simulink model "IEEE123bus_v2019b_Discrete_ZIPload"  (R2019b)
settings: Solver=ode4  StartTime=0.0  StopTime=5  FixedStep=Ts  MaxStep=1e-4  RelTol=1e-3
InitFcn:
  | a=1; % Loading Factor
  | Ts=50e-6;
  | % phase to sequence conversion of RXB matrices
  | c=1*exp(sqrt(-1)*(120*pi/180));
  | T=[1 1 1;1 c*c c;1 c c*c];
  | Tinv=1/3*[1 1 1;1 c c*c;1 c*c c];
  | 
  | % Simulation data for the IEEE 123 Node Test Feeder model
  | mi2km = 1.60934;%  miles to km conversion
  | ft2km = 0.0003048; % feet to km conversion
  | ms2F = 1*1e-6/(2*pi*60);% microsiemens to Farads conversion
  | 
  | %% Configuration 1
  | % Series Resitance and Reactance - ohm/mile
  | R_1 = [0.4576 0.1560 0.1535;0.1560 0.4666 0.1580;0.1535 0.1580 0.4615];
  | X_1 = [1.0780 0.5017 0.3849;0.5017 1.0482 0.4236;0.3849 0.4236 1.0651];
  | % charging susceptance - microsiemens/mile
  | B_1 = [5.6765 -1.8319 -0.6982;-1.8319 5.9809 -1.1645;-0.6982 -1.1645 5.3971];
  | 
  | R_1 = R_1/mi2km;
  | Rseq=Tinv*R_1*T;
  | R1_1=Rseq(2,2);R0_1=Rseq(1,1);
  | 
  | L_1 = (X_1/(2*pi*60))/mi2km;
  | Lseq=Tinv*L_1*T;
  | L1_1=Lseq(2,2);L0_1=Lseq(1,1);
  | 
  | C_1 =(B_1*ms2F)/mi2km;
  | Cseq=Tinv*C_1*T;
  | C1_1=Cseq(2,2);C0_1=Cseq(1,1);
  | %% Configuration 2 - series reactance - ohm/mile
  | R_2 = [0.4666 0.1580 0.1560;0.1580 0.4615 0.1535;0.1560 0.1535 0.4576];
  | X_2 = [1.0482 0.4236 0.5017;0.4236 1.0651 0.3849;0.5017 0.3849 1.0780];
  | % charging susceptance - microsiemens/mile
  | B_2 = [5.9809 -1.1645 -1.8319;-1.1645 5.3971 -0.6982;-1.8319 -0.6982 5.6765];
  | 
  | R_2 = R_2/mi2km;
  | Rseq=Tinv*R_2*T;
  | R1_2=Rseq(2,2);R0_2=Rseq(1,1);
  | 
  | L_2 = (X_2/(2*pi*60))/mi2km;
  | Lseq=Tinv*L_2*T;
  | L1_2=Lseq(2,2);L0_2=Lseq(1,1);
  | 
  | C_2 =(B_2*ms2F)/mi2km;
  | Cseq=Tinv*C_2*T;
  | C1_2=Cseq(2,2);C0_2=Cseq(1,1);
  | %% Configuration 3 - series reactance - ohm/mile
  | R_3 = [0.4615 0.1535 0.1580;0.1535 0.4576 0.1560;0.1580 0.1560 0.4666];
  | X_3 = [1.0651 0.3849 0.4236;0.3849 1.0780 0.5017;0.4236 0.5017 1.0482];
  | % charging susceptance - microsiemens/mile
  | B_3 = [5.3971 -0.6982 -1.1645;-0.6982 5.6765 -1.8319; -1.1645 -1.8319 5.9809];
  | 
  | R_3 = R_3/mi2km;
  | Rseq=Tinv*R_3*T;
  | R1_3=Rseq(2,2);R0_3=Rseq(1,1);
  | 
  | L_3 = (X_3/(2*pi*60))/mi2km;
  | Lseq=Tinv*L_3*T;
  | L1_3=Lseq(2,2);L0_3=Lseq(1,1);
  | ... (+157 lines)
undefined symbols (not defined in the file): D1, Delta, find_system
libraries: powerlib x971, powerlib_meascontrol x294
(part 14 of 14)

== matlab function IEEE123bus_v2019b_Discrete_ZIPload/55 Y Z/Embedded MATLAB Function ==
  data: Iinjinst output; Vmeas input; LoadType parameter; Vnom parameter; Pnom parameter; Qnom parameter; Vlim parameter; fnom parameter; clock input; Ddel input
%Single Phase ZIP Load
%Author: Arun Suresh, University of North Carolina, Charlotte
%Iinj=((Pnom+jQnom)/Vmeas)'
function Iinjinst = InjectedCurrent(Vmeas,LoadType,Vnom,Pnom,Qnom,Vlim,fnom,clock,Ddel)
% Calculate Pl and Ql.
%  Vmeas=1.2303e+03 + 1.9328e+03i;
Kz=0;Ki=0;Kp=0;
Vk=(abs(Vmeas)/Vnom);%(Vmeas/Vnom)
switch LoadType  % 1 for Constant Z, 2 for Constant I and 3 for Constant P, 
    case 1
        Kz=1;
    case 2
        if Vk >= Vlim % convert to Constant Z load due to voltage violation
            Ki=1;
        else
            Kz=1;
        end
    case 3
        if Vk >= Vlim % convert to Constant Z load due to voltage violation
           Kp=1;
        else
            Kz=1;
        end          
 
end
Pl=Pnom *((Kz*Vk*Vk)+(Ki*Vk)+(Kp));
Ql=Qnom *((Kz*Vk*Vk)+(Ki*Vk)+(Kp));
% Net Injected Curent.
% j=sqrt(-1);
Iinj = conj((Pl+j*Ql)/Vmeas);
Iinjinst =abs(Iinj)*sqrt(2)*sin(2*fnom*pi*clock + angle(Iinj)+Ddel);
yt=Iinj;

== matlab function IEEE123bus_v2019b_Discrete_ZIPload/64 Y I/Embedded MATLAB Function ==
  data: Iinjinst output; Vmeas input; LoadType parameter; Vnom parameter; Pnom parameter; Qnom parameter; Vlim parameter; fnom parameter; clock input; Ddel input
%Single Phase ZIP Load
%Author: Arun Suresh, University of North Carolina, Charlotte
%Iinj=((Pnom+jQnom)/Vmeas)'
function Iinjinst = InjectedCurrent(Vmeas,LoadType,Vnom,Pnom,Qnom,Vlim,fnom,clock,Ddel)
% Calculate Pl and Ql.
%  Vmeas=1.2303e+03 + 1.9328e+03i;
Kz=0;Ki=0;Kp=0;
Vk=(abs(Vmeas)/Vnom);%(Vmeas/Vnom)
switch LoadType  % 1 for Constant Z, 2 for Constant I and 3 for Constant P, 
    case 1
        Kz=1;
    case 2
        if Vk >= Vlim % convert to Constant Z load due to voltage violation
            Ki=1;
        else
            Kz=1;
        end
    case 3
        if Vk >= Vlim % convert to Constant Z load due to voltage violation
           Kp=1;
        else
            Kz=1;
        end          
 
end
Pl=Pnom *((Kz*Vk*Vk)+(Ki*Vk)+(Kp));
Ql=Qnom *((Kz*Vk*Vk)+(Ki*Vk)+(Kp));
% Net Injected Curent.
% j=sqrt(-1);
Iinj = conj((Pl+j*Ql)/Vmeas);
Iinjinst =abs(Iinj)*sqrt(2)*sin(2*fnom*pi*clock + angle(Iinj)+Ddel);
yt=Iinj;

== matlab function IEEE123bus_v2019b_Discrete_ZIPload/66 Y PQ/Embedded MATLAB Function ==
  data: Iinjinst output; Vmeas input; LoadType parameter; Vnom parameter; Pnom parameter; Qnom parameter; Vlim parameter; fnom parameter; clock input; Ddel input
%Single Phase ZIP Load
%Author: Arun Suresh, University of North Carolina, Charlotte
%Iinj=((Pnom+jQnom)/Vmeas)'
function Iinjinst = InjectedCurrent(Vmeas,LoadType,Vnom,Pnom,Qnom,Vlim,fnom,clock,Ddel)
% Calculate Pl and Ql.
%  Vmeas=1.2303e+03 + 1.9328e+03i;
Kz=0;Ki=0;Kp=0;
Vk=(abs(Vmeas)/Vnom);%(Vmeas/Vnom)
switch LoadType  % 1 for Constant Z, 2 for Constant I and 3 for Constant P, 
    case 1
        Kz=1;
    case 2
        if Vk >= Vlim % convert to Constant Z load due to voltage violation
            Ki=1;
        else
            Kz=1;
        end
    case 3
        if Vk >= Vlim % convert to Constant Z load due to voltage violation
           Kp=1;
        else
            Kz=1;
        end          
 
end
Pl=Pnom *((Kz*Vk*Vk)+(Ki*Vk)+(Kp));
Ql=Qnom *((Kz*Vk*Vk)+(Ki*Vk)+(Kp));
% Net Injected Curent.
% j=sqrt(-1);
Iinj = conj((Pl+j*Ql)/Vmeas);
Iinjinst =abs(Iinj)*sqrt(2)*sin(2*fnom*pi*clock + angle(Iinj)+Ddel);
yt=Iinj;

== matlab function IEEE123bus_v2019b_Discrete_ZIPload/96 Y PQ/Embedded MATLAB Function ==
  data: Iinjinst output; Vmeas input; LoadType parameter; Vnom parameter; Pnom parameter; Qnom parameter; Vlim parameter; fnom parameter; clock input; Ddel input
%Single Phase ZIP Load
%Author: Arun Suresh, University of North Carolina, Charlotte
%Iinj=((Pnom+jQnom)/Vmeas)'
function Iinjinst = InjectedCurrent(Vmeas,LoadType,Vnom,Pnom,Qnom,Vlim,fnom,clock,Ddel)
% Calculate Pl and Ql.
%  Vmeas=1.2303e+03 + 1.9328e+03i;
Kz=0;Ki=0;Kp=0;
Vk=(abs(Vmeas)/Vnom);%(Vmeas/Vnom)
switch LoadType  % 1 for Constant Z, 2 for Constant I and 3 for Constant P, 
    case 1
        Kz=1;
    case 2
        if Vk >= Vlim % convert to Constant Z load due to voltage violation
            Ki=1;
        else
            Kz=1;
        end
    case 3
        if Vk >= Vlim % convert to Constant Z load due to voltage violation
           Kp=1;
        else
            Kz=1;
        end          
 
end
Pl=Pnom *((Kz*Vk*Vk)+(Ki*Vk)+(Kp));
Ql=Qnom *((Kz*Vk*Vk)+(Ki*Vk)+(Kp));
% Net Injected Curent.
% j=sqrt(-1);
Iinj = conj((Pl+j*Ql)/Vmeas);
Iinjinst =abs(Iinj)*sqrt(2)*sin(2*fnom*pi*clock + angle(Iinj)+Ddel);
yt=Iinj;

== matlab function IEEE123bus_v2019b_Discrete_ZIPload/95 Y PQ/Embedded MATLAB Function ==
  data: Iinjinst output; Vmeas input; LoadType parameter; Vnom parameter; Pnom parameter; Qnom parameter; Vlim parameter; fnom parameter; clock input; Ddel input
%Single Phase ZIP Load
%Author: Arun Suresh, University of North Carolina, Charlotte
%Iinj=((Pnom+jQnom)/Vmeas)'
function Iinjinst = InjectedCurrent(Vmeas,LoadType,Vnom,Pnom,Qnom,Vlim,fnom,clock,Ddel)
% Calculate Pl and Ql.
%  Vmeas=1.2303e+03 + 1.9328e+03i;
Kz=0;Ki=0;Kp=0;
Vk=(abs(Vmeas)/Vnom);%(Vmeas/Vnom)
switch LoadType  % 1 for Constant Z, 2 for Constant I and 3 for Constant P, 
    case 1
        Kz=1;
    case 2
        if Vk >= Vlim % convert to Constant Z load due to voltage violation
            Ki=1;
        else
            Kz=1;
        end
    case 3
        if Vk >= Vlim % convert to Constant Z load due to voltage violation
           Kp=1;
        else
            Kz=1;
        end          
 
end
Pl=Pnom *((Kz*Vk*Vk)+(Ki*Vk)+(Kp));
Ql=Qnom *((Kz*Vk*Vk)+(Ki*Vk)+(Kp));
% Net Injected Curent.
% j=sqrt(-1);
Iinj = conj((Pl+j*Ql)/Vmeas);
Iinjinst =abs(Iinj)*sqrt(2)*sin(2*fnom*pi*clock + angle(Iinj)+Ddel);
yt=Iinj;

== matlab function IEEE123bus_v2019b_Discrete_ZIPload/111 Y PQ/Embedded MATLAB Function ==
  data: Iinjinst output; Vmeas input; LoadType parameter; Vnom parameter; Pnom parameter; Qnom parameter; Vlim parameter; fnom parameter; clock input; Ddel input
%Single Phase ZIP Load
%Author: Arun Suresh, University of North Carolina, Charlotte
%Iinj=((Pnom+jQnom)/Vmeas)'
function Iinjinst = InjectedCurrent(Vmeas,LoadType,Vnom,Pnom,Qnom,Vlim,fnom,clock,Ddel)
% Calculate Pl and Ql.
%  Vmeas=1.2303e+03 + 1.9328e+03i;
Kz=0;Ki=0;Kp=0;
Vk=(abs(Vmeas)/Vnom);%(Vmeas/Vnom)
switch LoadType  % 1 for Constant Z, 2 for Constant I and 3 for Constant P, 
    case 1
        Kz=1;
    case 2
        if Vk >= Vlim % convert to Constant Z load due to voltage violation
            Ki=1;
        else
            Kz=1;
        end
    case 3
        if Vk >= Vlim % convert to Constant Z load due to voltage violation
           Kp=1;
        else
            Kz=1;
        end          
 
end
Pl=Pnom *((Kz*Vk*Vk)+(Ki*Vk)+(Kp));
Ql=Qnom *((Kz*Vk*Vk)+(Ki*Vk)+(Kp));
% Net Injected Curent.
% j=sqrt(-1);
Iinj = conj((Pl+j*Ql)/Vmeas);
Iinjinst =abs(Iinj)*sqrt(2)*sin(2*fnom*pi*clock + angle(Iinj)+Ddel);
yt=Iinj;

== matlab function IEEE123bus_v2019b_Discrete_ZIPload/109 Y PQ/Embedded MATLAB Function ==
  data: Iinjinst output; Vmeas input; LoadType parameter; Vnom parameter; Pnom parameter; Qnom parameter; Vlim parameter; fnom parameter; clock input; Ddel input
%Single Phase ZIP Load
%Author: Arun Suresh, University of North Carolina, Charlotte
%Iinj=((Pnom+jQnom)/Vmeas)'
function Iinjinst = InjectedCurrent(Vmeas,LoadType,Vnom,Pnom,Qnom,Vlim,fnom,clock,Ddel)
% Calculate Pl and Ql.
%  Vmeas=1.2303e+03 + 1.9328e+03i;
Kz=0;Ki=0;Kp=0;
Vk=(abs(Vmeas)/Vnom);%(Vmeas/Vnom)
switch LoadType  % 1 for Constant Z, 2 for Constant I and 3 for Constant P, 
    case 1
        Kz=1;
    case 2
        if Vk >= Vlim % convert to Constant Z load due to voltage violation
            Ki=1;
        else
            Kz=1;
        end
    case 3
        if Vk >= Vlim % convert to Constant Z load due to voltage violation
           Kp=1;
        else
            Kz=1;
        end          
 
end
Pl=Pnom *((Kz*Vk*Vk)+(Ki*Vk)+(Kp));
Ql=Qnom *((Kz*Vk*Vk)+(Ki*Vk)+(Kp));
% Net Injected Curent.
% j=sqrt(-1);
Iinj = conj((Pl+j*Ql)/Vmeas);
Iinjinst =abs(Iinj)*sqrt(2)*sin(2*fnom*pi*clock + angle(Iinj)+Ddel);
yt=Iinj;

== matlab function IEEE123bus_v2019b_Discrete_ZIPload/114 Y PQ/Embedded MATLAB Function ==
  data: Iinjinst output; Vmeas input; LoadType parameter; Vnom parameter; Pnom parameter; Qnom parameter; Vlim parameter; fnom parameter; clock input; Ddel input
%Single Phase ZIP Load
%Author: Arun Suresh, University of North Carolina, Charlotte
%Iinj=((Pnom+jQnom)/Vmeas)'
function Iinjinst = InjectedCurrent(Vmeas,LoadType,Vnom,Pnom,Qnom,Vlim,fnom,clock,Ddel)
% Calculate Pl and Ql.
%  Vmeas=1.2303e+03 + 1.9328e+03i;
Kz=0;Ki=0;Kp=0;
Vk=(abs(Vmeas)/Vnom);%(Vmeas/Vnom)
switch LoadType  % 1 for Constant Z, 2 for Constant I and 3 for Constant P, 
    case 1
        Kz=1;
    case 2
        if Vk >= Vlim % convert to Constant Z load due to voltage violation
            Ki=1;
        else
            Kz=1;
        end
    case 3
        if Vk >= Vlim % convert to Constant Z load due to voltage violation
           Kp=1;
        else
            Kz=1;
        end          
 
end
Pl=Pnom *((Kz*Vk*Vk)+(Ki*Vk)+(Kp));
Ql=Qnom *((Kz*Vk*Vk)+(Ki*Vk)+(Kp));
% Net Injected Curent.
% j=sqrt(-1);
Iinj = conj((Pl+j*Ql)/Vmeas);
Iinjinst =abs(Iinj)*sqrt(2)*sin(2*fnom*pi*clock + angle(Iinj)+Ddel);
yt=Iinj;

== matlab function IEEE123bus_v2019b_Discrete_ZIPload/113 Y Z/Embedded MATLAB Function ==
  data: Iinjinst output; Vmeas input; LoadType parameter; Vnom parameter; Pnom parameter; Qnom parameter; Vlim parameter; fnom parameter; clock input; Ddel input
%Single Phase ZIP Load
%Author: Arun Suresh, University of North Carolina, Charlotte
%Iinj=((Pnom+jQnom)/Vmeas)'
function Iinjinst = InjectedCurrent(Vmeas,LoadType,Vnom,Pnom,Qnom,Vlim,fnom,clock,Ddel)
% Calculate Pl and Ql.
%  Vmeas=1.2303e+03 + 1.9328e+03i;
Kz=0;Ki=0;Kp=0;
Vk=(abs(Vmeas)/Vnom);%(Vmeas/Vnom)
switch LoadType  % 1 for Constant Z, 2 for Constant I and 3 for Constant P, 
    case 1
        Kz=1;
    case 2
        if Vk >= Vlim % convert to Constant Z load due to voltage violation
            Ki=1;
        else
            Kz=1;
        end
    case 3
        if Vk >= Vlim % convert to Constant Z load due to voltage violation
           Kp=1;
        else
            Kz=1;
        end          
 
end
Pl=Pnom *((Kz*Vk*Vk)+(Ki*Vk)+(Kp));
Ql=Qnom *((Kz*Vk*Vk)+(Ki*Vk)+(Kp));
% Net Injected Curent.
% j=sqrt(-1);
Iinj = conj((Pl+j*Ql)/Vmeas);
Iinjinst =abs(Iinj)*sqrt(2)*sin(2*fnom*pi*clock + angle(Iinj)+Ddel);
yt=Iinj;

== matlab function IEEE123bus_v2019b_Discrete_ZIPload/112 Y I/Embedded MATLAB Function ==
  data: Iinjinst output; Vmeas input; LoadType parameter; Vnom parameter; Pnom parameter; Qnom parameter; Vlim parameter; fnom parameter; clock input; Ddel input
%Single Phase ZIP Load
%Author: Arun Suresh, University of North Carolina, Charlotte
%Iinj=((Pnom+jQnom)/Vmeas)'
function Iinjinst = InjectedCurrent(Vmeas,LoadType,Vnom,Pnom,Qnom,Vlim,fnom,clock,Ddel)
% Calculate Pl and Ql.
%  Vmeas=1.2303e+03 + 1.9328e+03i;
Kz=0;Ki=0;Kp=0;
Vk=(abs(Vmeas)/Vnom);%(Vmeas/Vnom)
switch LoadType  % 1 for Constant Z, 2 for Constant I and 3 for Constant P, 
    case 1
        Kz=1;
    case 2
        if Vk >= Vlim % convert to Constant Z load due to voltage violation
            Ki=1;
        else
            Kz=1;
        end
    case 3
        if Vk >= Vlim % convert to Constant Z load due to voltage violation
           Kp=1;
        else
            Kz=1;
        end          
 
end
Pl=Pnom *((Kz*Vk*Vk)+(Ki*Vk)+(Kp));
Ql=Qnom *((Kz*Vk*Vk)+(Ki*Vk)+(Kp));
% Net Injected Curent.
% j=sqrt(-1);
Iinj = conj((Pl+j*Ql)/Vmeas);
Iinjinst =abs(Iinj)*sqrt(2)*sin(2*fnom*pi*clock + angle(Iinj)+Ddel);
yt=Iinj;

== matlab function IEEE123bus_v2019b_Discrete_ZIPload/106 Y PQ/Embedded MATLAB Function ==
  data: Iinjinst output; Vmeas input; LoadType parameter; Vnom parameter; Pnom parameter; Qnom parameter; Vlim parameter; fnom parameter; clock input; Ddel input
%Single Phase ZIP Load
%Author: Arun Suresh, University of North Carolina, Charlotte
%Iinj=((Pnom+jQnom)/Vmeas)'
function Iinjinst = InjectedCurrent(Vmeas,LoadType,Vnom,Pnom,Qnom,Vlim,fnom,clock,Ddel)
% Calculate Pl and Ql.
%  Vmeas=1.2303e+03 + 1.9328e+03i;
Kz=0;Ki=0;Kp=0;
Vk=(abs(Vmeas)/Vnom);%(Vmeas/Vnom)
switch LoadType  % 1 for Constant Z, 2 for Constant I and 3 for Constant P, 
    case 1
        Kz=1;
    case 2
        if Vk >= Vlim % convert to Constant Z load due to voltage violation
            Ki=1;
        else
            Kz=1;
        end
    case 3
        if Vk >= Vlim % convert to Constant Z load due to voltage violation
           Kp=1;
        else
            Kz=1;
        end          
 
end
Pl=Pnom *((Kz*Vk*Vk)+(Ki*Vk)+(Kp));
Ql=Qnom *((Kz*Vk*Vk)+(Ki*Vk)+(Kp));
% Net Injected Curent.
% j=sqrt(-1);
Iinj = conj((Pl+j*Ql)/Vmeas);
Iinjinst =abs(Iinj)*sqrt(2)*sin(2*fnom*pi*clock + angle(Iinj)+Ddel);
yt=Iinj;

== matlab function IEEE123bus_v2019b_Discrete_ZIPload/107 Y PQ/Embedded MATLAB Function ==
  data: Iinjinst output; Vmeas input; LoadType parameter; Vnom parameter; Pnom parameter; Qnom parameter; Vlim parameter; fnom parameter; clock input; Ddel input
%Single Phase ZIP Load
%Author: Arun Suresh, University of North Carolina, Charlotte
%Iinj=((Pnom+jQnom)/Vmeas)'
function Iinjinst = InjectedCurrent(Vmeas,LoadType,Vnom,Pnom,Qnom,Vlim,fnom,clock,Ddel)
% Calculate Pl and Ql.
%  Vmeas=1.2303e+03 + 1.9328e+03i;
Kz=0;Ki=0;Kp=0;
Vk=(abs(Vmeas)/Vnom);%(Vmeas/Vnom)
switch LoadType  % 1 for Constant Z, 2 for Constant I and 3 for Constant P, 
    case 1
        Kz=1;
    case 2
        if Vk >= Vlim % convert to Constant Z load due to voltage violation
            Ki=1;
        else
            Kz=1;
        end
    case 3
        if Vk >= Vlim % convert to Constant Z load due to voltage violation
           Kp=1;
        else
            Kz=1;
        end          
 
end
Pl=Pnom *((Kz*Vk*Vk)+(Ki*Vk)+(Kp));
Ql=Qnom *((Kz*Vk*Vk)+(Ki*Vk)+(Kp));
% Net Injected Curent.
% j=sqrt(-1);
Iinj = conj((Pl+j*Ql)/Vmeas);
Iinjinst =abs(Iinj)*sqrt(2)*sin(2*fnom*pi*clock + angle(Iinj)+Ddel);
yt=Iinj;

== matlab function IEEE123bus_v2019b_Discrete_ZIPload/103 Y PQ/Embedded MATLAB Function ==
  data: Iinjinst output; Vmeas input; LoadType parameter; Vnom parameter; Pnom parameter; Qnom parameter; Vlim parameter; fnom parameter; clock input; Ddel input
%Single Phase ZIP Load
%Author: Arun Suresh, University of North Carolina, Charlotte
%Iinj=((Pnom+jQnom)/Vmeas)'
function Iinjinst = InjectedCurrent(Vmeas,LoadType,Vnom,Pnom,Qnom,Vlim,fnom,clock,Ddel)
% Calculate Pl and Ql.
%  Vmeas=1.2303e+03 + 1.9328e+03i;
Kz=0;Ki=0;Kp=0;
Vk=(abs(Vmeas)/Vnom);%(Vmeas/Vnom)
switch LoadType  % 1 for Constant Z, 2 for Constant I and 3 for Constant P, 
    case 1
        Kz=1;
    case 2
        if Vk >= Vlim % convert to Constant Z load due to voltage violation
            Ki=1;
        else
            Kz=1;
        end
    case 3
        if Vk >= Vlim % convert to Constant Z load due to voltage violation
           Kp=1;
        else
            Kz=1;
        end          
 
end
Pl=Pnom *((Kz*Vk*Vk)+(Ki*Vk)+(Kp));
Ql=Qnom *((Kz*Vk*Vk)+(Ki*Vk)+(Kp));
% Net Injected Curent.
% j=sqrt(-1);
Iinj = conj((Pl+j*Ql)/Vmeas);
Iinjinst =abs(Iinj)*sqrt(2)*sin(2*fnom*pi*clock + angle(Iinj)+Ddel);
yt=Iinj;

== matlab function IEEE123bus_v2019b_Discrete_ZIPload/104 Y PQ/Embedded MATLAB Function ==
  data: Iinjinst output; Vmeas input; LoadType parameter; Vnom parameter; Pnom parameter; Qnom parameter; Vlim parameter; fnom parameter; clock input; Ddel input
%Single Phase ZIP Load
%Author: Arun Suresh, University of North Carolina, Charlotte
%Iinj=((Pnom+jQnom)/Vmeas)'
function Iinjinst = InjectedCurrent(Vmeas,LoadType,Vnom,Pnom,Qnom,Vlim,fnom,clock,Ddel)
% Calculate Pl and Ql.
%  Vmeas=1.2303e+03 + 1.9328e+03i;
Kz=0;Ki=0;Kp=0;
Vk=(abs(Vmeas)/Vnom);%(Vmeas/Vnom)
switch LoadType  % 1 for Constant Z, 2 for Constant I and 3 for Constant P, 
    case 1
        Kz=1;
    case 2
        if Vk >= Vlim % convert to Constant Z load due to voltage violation
            Ki=1;
        else
            Kz=1;
        end
    case 3
        if Vk >= Vlim % convert to Constant Z load due to voltage violation
           Kp=1;
        else
            Kz=1;
        end          
 
end
Pl=Pnom *((Kz*Vk*Vk)+(Ki*Vk)+(Kp));
Ql=Qnom *((Kz*Vk*Vk)+(Ki*Vk)+(Kp));
% Net Injected Curent.
% j=sqrt(-1);
Iinj = conj((Pl+j*Ql)/Vmeas);
Iinjinst =abs(Iinj)*sqrt(2)*sin(2*fnom*pi*clock + angle(Iinj)+Ddel);
yt=Iinj;

== matlab function IEEE123bus_v2019b_Discrete_ZIPload/102 Y PQ/Embedded MATLAB Function ==
  data: Iinjinst output; Vmeas input; LoadType parameter; Vnom parameter; Pnom parameter; Qnom parameter; Vlim parameter; fnom parameter; clock input; Ddel input
%Single Phase ZIP Load
%Author: Arun Suresh, University of North Carolina, Charlotte
%Iinj=((Pnom+jQnom)/Vmeas)'
function Iinjinst = InjectedCurrent(Vmeas,LoadType,Vnom,Pnom,Qnom,Vlim,fnom,clock,Ddel)
% Calculate Pl and Ql.
%  Vmeas=1.2303e+03 + 1.9328e+03i;
Kz=0;Ki=0;Kp=0;
Vk=(abs(Vmeas)/Vnom);%(Vmeas/Vnom)
switch LoadType  % 1 for Constant Z, 2 for Constant I and 3 for Constant P, 
    case 1
        Kz=1;
    case 2
        if Vk >= Vlim % convert to Constant Z load due to voltage violation
            Ki=1;
        else
            Kz=1;
        end
    case 3
        if Vk >= Vlim % convert to Constant Z load due to voltage violation
           Kp=1;
        else
            Kz=1;
        end          
 
end
Pl=Pnom *((Kz*Vk*Vk)+(Ki*Vk)+(Kp));
Ql=Qnom *((Kz*Vk*Vk)+(Ki*Vk)+(Kp));
% Net Injected Curent.
% j=sqrt(-1);
Iinj = conj((Pl+j*Ql)/Vmeas);
Iinjinst =abs(Iinj)*sqrt(2)*sin(2*fnom*pi*clock + angle(Iinj)+Ddel);
yt=Iinj;

== matlab function IEEE123bus_v2019b_Discrete_ZIPload/98 Y PQ/Embedded MATLAB Function ==
  data: Iinjinst output; Vmeas input; LoadType parameter; Vnom parameter; Pnom parameter; Qnom parameter; Vlim parameter; fnom parameter; clock input; Ddel input
%Single Phase ZIP Load
%Author: Arun Suresh, University of North Carolina, Charlotte
%Iinj=((Pnom+jQnom)/Vmeas)'
function Iinjinst = InjectedCurrent(Vmeas,LoadType,Vnom,Pnom,Qnom,Vlim,fnom,clock,Ddel)
% Calculate Pl and Ql.
%  Vmeas=1.2303e+03 + 1.9328e+03i;
Kz=0;Ki=0;Kp=0;
Vk=(abs(Vmeas)/Vnom);%(Vmeas/Vnom)
switch LoadType  % 1 for Constant Z, 2 for Constant I and 3 for Constant P, 
    case 1
        Kz=1;
    case 2
        if Vk >= Vlim % convert to Constant Z load due to voltage violation
            Ki=1;
        else
            Kz=1;
        end
    case 3
        if Vk >= Vlim % convert to Constant Z load due to voltage violation
           Kp=1;
        else
            Kz=1;
        end          
 
end
Pl=Pnom *((Kz*Vk*Vk)+(Ki*Vk)+(Kp));
Ql=Qnom *((Kz*Vk*Vk)+(Ki*Vk)+(Kp));
% Net Injected Curent.
% j=sqrt(-1);
Iinj = conj((Pl+j*Ql)/Vmeas);
Iinjinst =abs(Iinj)*sqrt(2)*sin(2*fnom*pi*clock + angle(Iinj)+Ddel);
yt=Iinj;

== matlab function IEEE123bus_v2019b_Discrete_ZIPload/99 Y PQ/Embedded MATLAB Function ==
  data: Iinjinst output; Vmeas input; LoadType parameter; Vnom parameter; Pnom parameter; Qnom parameter; Vlim parameter; fnom parameter; clock input; Ddel input
%Single Phase ZIP Load
%Author: Arun Suresh, University of North Carolina, Charlotte
%Iinj=((Pnom+jQnom)/Vmeas)'
function Iinjinst = InjectedCurrent(Vmeas,LoadType,Vnom,Pnom,Qnom,Vlim,fnom,clock,Ddel)
% Calculate Pl and Ql.
%  Vmeas=1.2303e+03 + 1.9328e+03i;
Kz=0;Ki=0;Kp=0;
Vk=(abs(Vmeas)/Vnom);%(Vmeas/Vnom)
switch LoadType  % 1 for Constant Z, 2 for Constant I and 3 for Constant P, 
    case 1
        Kz=1;
    case 2
        if Vk >= Vlim % convert to Constant Z load due to voltage violation
            Ki=1;
        else
            Kz=1;
        end
    case 3
        if Vk >= Vlim % convert to Constant Z load due to voltage violation
           Kp=1;
        else
            Kz=1;
        end          
 
end
Pl=Pnom *((Kz*Vk*Vk)+(Ki*Vk)+(Kp));
Ql=Qnom *((Kz*Vk*Vk)+(Ki*Vk)+(Kp));
% Net Injected Curent.
% j=sqrt(-1);
Iinj = conj((Pl+j*Ql)/Vmeas);
Iinjinst =abs(Iinj)*sqrt(2)*sin(2*fnom*pi*clock + angle(Iinj)+Ddel);
yt=Iinj;

== matlab function IEEE123bus_v2019b_Discrete_ZIPload/100 Y Z/Embedded MATLAB Function ==
  data: Iinjinst output; Vmeas input; LoadType parameter; Vnom parameter; Pnom parameter; Qnom parameter; Vlim parameter; fnom parameter; clock input; Ddel input
%Single Phase ZIP Load
%Author: Arun Suresh, University of North Carolina, Charlotte
%Iinj=((Pnom+jQnom)/Vmeas)'
function Iinjinst = InjectedCurrent(Vmeas,LoadType,Vnom,Pnom,Qnom,Vlim,fnom,clock,Ddel)
% Calculate Pl and Ql.
%  Vmeas=1.2303e+03 + 1.9328e+03i;
Kz=0;Ki=0;Kp=0;
Vk=(abs(Vmeas)/Vnom);%(Vmeas/Vnom)
switch LoadType  % 1 for Constant Z, 2 for Constant I and 3 for Constant P, 
    case 1
        Kz=1;
    case 2
        if Vk >= Vlim % convert to Constant Z load due to voltage violation
            Ki=1;
        else
            Kz=1;
        end
    case 3
        if Vk >= Vlim % convert to Constant Z load due to voltage violation
           Kp=1;
        else
            Kz=1;
        end          
 
end
Pl=Pnom *((Kz*Vk*Vk)+(Ki*Vk)+(Kp));
Ql=Qnom *((Kz*Vk*Vk)+(Ki*Vk)+(Kp));
% Net Injected Curent.
% j=sqrt(-1);
Iinj = conj((Pl+j*Ql)/Vmeas);
Iinjinst =abs(Iinj)*sqrt(2)*sin(2*fnom*pi*clock + angle(Iinj)+Ddel);
yt=Iinj;

== matlab function IEEE123bus_v2019b_Discrete_ZIPload/71 Y PQ/Embedded MATLAB Function ==
  data: Iinjinst output; Vmeas input; LoadType parameter; Vnom parameter; Pnom parameter; Qnom parameter; Vlim parameter; fnom parameter; clock input; Ddel input
%Single Phase ZIP Load
%Author: Arun Suresh, University of North Carolina, Charlotte
%Iinj=((Pnom+jQnom)/Vmeas)'
function Iinjinst = InjectedCurrent(Vmeas,LoadType,Vnom,Pnom,Qnom,Vlim,fnom,clock,Ddel)
% Calculate Pl and Ql.
%  Vmeas=1.2303e+03 + 1.9328e+03i;
Kz=0;Ki=0;Kp=0;
Vk=(abs(Vmeas)/Vnom);%(Vmeas/Vnom)
switch LoadType  % 1 for Constant Z, 2 for Constant I and 3 for Constant P, 
    case 1
        Kz=1;
    case 2
        if Vk >= Vlim % convert to Constant Z load due to voltage violation
            Ki=1;
        else
            Kz=1;
        end
    case 3
        if Vk >= Vlim % convert to Constant Z load due to voltage violation
           Kp=1;
        else
            Kz=1;
        end          
 
end
Pl=Pnom *((Kz*Vk*Vk)+(Ki*Vk)+(Kp));
Ql=Qnom *((Kz*Vk*Vk)+(Ki*Vk)+(Kp));
% Net Injected Curent.
% j=sqrt(-1);
Iinj = conj((Pl+j*Ql)/Vmeas);
Iinjinst =abs(Iinj)*sqrt(2)*sin(2*fnom*pi*clock + angle(Iinj)+Ddel);
yt=Iinj;

== matlab function IEEE123bus_v2019b_Discrete_ZIPload/69 Y PQ/Embedded MATLAB Function ==
  data: Iinjinst output; Vmeas input; LoadType parameter; Vnom parameter; Pnom parameter; Qnom parameter; Vlim parameter; fnom parameter; clock input; Ddel input
%Single Phase ZIP Load
%Author: Arun Suresh, University of North Carolina, Charlotte
%Iinj=((Pnom+jQnom)/Vmeas)'
function Iinjinst = InjectedCurrent(Vmeas,LoadType,Vnom,Pnom,Qnom,Vlim,fnom,clock,Ddel)
% Calculate Pl and Ql.
%  Vmeas=1.2303e+03 + 1.9328e+03i;
Kz=0;Ki=0;Kp=0;
Vk=(abs(Vmeas)/Vnom);%(Vmeas/Vnom)
switch LoadType  % 1 for Constant Z, 2 for Constant I and 3 for Constant P, 
    case 1
        Kz=1;
    case 2
        if Vk >= Vlim % convert to Constant Z load due to voltage violation
            Ki=1;
        else
            Kz=1;
        end
    case 3
        if Vk >= Vlim % convert to Constant Z load due to voltage violation
           Kp=1;
        else
            Kz=1;
        end          
 
end
Pl=Pnom *((Kz*Vk*Vk)+(Ki*Vk)+(Kp));
Ql=Qnom *((Kz*Vk*Vk)+(Ki*Vk)+(Kp));
% Net Injected Curent.
% j=sqrt(-1);
Iinj = conj((Pl+j*Ql)/Vmeas);
Iinjinst =abs(Iinj)*sqrt(2)*sin(2*fnom*pi*clock + angle(Iinj)+Ddel);
yt=Iinj;

== matlab function IEEE123bus_v2019b_Discrete_ZIPload/68 Y PQ/Embedded MATLAB Function ==
  data: Iinjinst output; Vmeas input; LoadType parameter; Vnom parameter; Pnom parameter; Qnom parameter; Vlim parameter; fnom parameter; clock input; Ddel input
%Single Phase ZIP Load
%Author: Arun Suresh, University of North Carolina, Charlotte
%Iinj=((Pnom+jQnom)/Vmeas)'
function Iinjinst = InjectedCurrent(Vmeas,LoadType,Vnom,Pnom,Qnom,Vlim,fnom,clock,Ddel)
% Calculate Pl and Ql.
%  Vmeas=1.2303e+03 + 1.9328e+03i;
Kz=0;Ki=0;Kp=0;
Vk=(abs(Vmeas)/Vnom);%(Vmeas/Vnom)
switch LoadType  % 1 for Constant Z, 2 for Constant I and 3 for Constant P, 
    case 1
        Kz=1;
    case 2
        if Vk >= Vlim % convert to Constant Z load due to voltage violation
            Ki=1;
        else
            Kz=1;
        end
    case 3
        if Vk >= Vlim % convert to Constant Z load due to voltage violation
           Kp=1;
        else
            Kz=1;
        end          
 
end
Pl=Pnom *((Kz*Vk*Vk)+(Ki*Vk)+(Kp));
Ql=Qnom *((Kz*Vk*Vk)+(Ki*Vk)+(Kp));
% Net Injected Curent.
% j=sqrt(-1);
Iinj = conj((Pl+j*Ql)/Vmeas);
Iinjinst =abs(Iinj)*sqrt(2)*sin(2*fnom*pi*clock + angle(Iinj)+Ddel);
yt=Iinj;

== matlab function IEEE123bus_v2019b_Discrete_ZIPload/70 Y PQ/Embedded MATLAB Function ==
  data: Iinjinst output; Vmeas input; LoadType parameter; Vnom parameter; Pnom parameter; Qnom parameter; Vlim parameter; fnom parameter; clock input; Ddel input
%Single Phase ZIP Load
%Author: Arun Suresh, University of North Carolina, Charlotte
%Iinj=((Pnom+jQnom)/Vmeas)'
function Iinjinst = InjectedCurrent(Vmeas,LoadType,Vnom,Pnom,Qnom,Vlim,fnom,clock,Ddel)
% Calculate Pl and Ql.
%  Vmeas=1.2303e+03 + 1.9328e+03i;
Kz=0;Ki=0;Kp=0;
Vk=(abs(Vmeas)/Vnom);%(Vmeas/Vnom)
switch LoadType  % 1 for Constant Z, 2 for Constant I and 3 for Constant P, 
    case 1
        Kz=1;
    case 2
        if Vk >= Vlim % convert to Constant Z load due to voltage violation
            Ki=1;
        else
            Kz=1;
        end
    case 3
        if Vk >= Vlim % convert to Constant Z load due to voltage violation
           Kp=1;
        else
            Kz=1;
        end          
 
end
Pl=Pnom *((Kz*Vk*Vk)+(Ki*Vk)+(Kp));
Ql=Qnom *((Kz*Vk*Vk)+(Ki*Vk)+(Kp));
% Net Injected Curent.
% j=sqrt(-1);
Iinj = conj((Pl+j*Ql)/Vmeas);
Iinjinst =abs(Iinj)*sqrt(2)*sin(2*fnom*pi*clock + angle(Iinj)+Ddel);
yt=Iinj;

== matlab function IEEE123bus_v2019b_Discrete_ZIPload/73 Y PQ/Embedded MATLAB Function ==
  data: Iinjinst output; Vmeas input; LoadType parameter; Vnom parameter; Pnom parameter; Qnom parameter; Vlim parameter; fnom parameter; clock input; Ddel input
%Single Phase ZIP Load
%Author: Arun Suresh, University of North Carolina, Charlotte
%Iinj=((Pnom+jQnom)/Vmeas)'
function Iinjinst = InjectedCurrent(Vmeas,LoadType,Vnom,Pnom,Qnom,Vlim,fnom,clock,Ddel)
% Calculate Pl and Ql.
%  Vmeas=1.2303e+03 + 1.9328e+03i;
Kz=0;Ki=0;Kp=0;
Vk=(abs(Vmeas)/Vnom);%(Vmeas/Vnom)
switch LoadType  % 1 for Constant Z, 2 for Constant I and 3 for Constant P, 
    case 1
        Kz=1;
    case 2
        if Vk >= Vlim % convert to Constant Z load due to voltage violation
            Ki=1;
        else
            Kz=1;
        end
    case 3
        if Vk >= Vlim % convert to Constant Z load due to voltage violation
           Kp=1;
        else
            Kz=1;
        end          
 
end
Pl=Pnom *((Kz*Vk*Vk)+(Ki*Vk)+(Kp));
Ql=Qnom *((Kz*Vk*Vk)+(Ki*Vk)+(Kp));
% Net Injected Curent.
% j=sqrt(-1);
Iinj = conj((Pl+j*Ql)/Vmeas);
Iinjinst =abs(Iinj)*sqrt(2)*sin(2*fnom*pi*clock + angle(Iinj)+Ddel);
yt=Iinj;

== matlab function IEEE123bus_v2019b_Discrete_ZIPload/75 Y PQ/Embedded MATLAB Function ==
  data: Iinjinst output; Vmeas input; LoadType parameter; Vnom parameter; Pnom parameter; Qnom parameter; Vlim parameter; fnom parameter; clock input; Ddel input
%Single Phase ZIP Load
%Author: Arun Suresh, University of North Carolina, Charlotte
%Iinj=((Pnom+jQnom)/Vmeas)'
function Iinjinst = InjectedCurrent(Vmeas,LoadType,Vnom,Pnom,Qnom,Vlim,fnom,clock,Ddel)
% Calculate Pl and Ql.
%  Vmeas=1.2303e+03 + 1.9328e+03i;
Kz=0;Ki=0;Kp=0;
Vk=(abs(Vmeas)/Vnom);%(Vmeas/Vnom)
switch LoadType  % 1 for Constant Z, 2 for Constant I and 3 for Constant P, 
    case 1
        Kz=1;
    case 2
        if Vk >= Vlim % convert to Constant Z load due to voltage violation
            Ki=1;
        else
            Kz=1;
        end
    case 3
        if Vk >= Vlim % convert to Constant Z load due to voltage violation
           Kp=1;
        else
            Kz=1;
        end          
 
end
Pl=Pnom *((Kz*Vk*Vk)+(Ki*Vk)+(Kp));
Ql=Qnom *((Kz*Vk*Vk)+(Ki*Vk)+(Kp));
% Net Injected Curent.
% j=sqrt(-1);
Iinj = conj((Pl+j*Ql)/Vmeas);
Iinjinst =abs(Iinj)*sqrt(2)*sin(2*fnom*pi*clock + angle(Iinj)+Ddel);
yt=Iinj;

== matlab function IEEE123bus_v2019b_Discrete_ZIPload/74 Y Z/Embedded MATLAB Function ==
  data: Iinjinst output; Vmeas input; LoadType parameter; Vnom parameter; Pnom parameter; Qnom parameter; Vlim parameter; fnom parameter; clock input; Ddel input
%Single Phase ZIP Load
%Author: Arun Suresh, University of North Carolina, Charlotte
%Iinj=((Pnom+jQnom)/Vmeas)'
function Iinjinst = InjectedCurrent(Vmeas,LoadType,Vnom,Pnom,Qnom,Vlim,fnom,clock,Ddel)
% Calculate Pl and Ql.
%  Vmeas=1.2303e+03 + 1.9328e+03i;
Kz=0;Ki=0;Kp=0;
Vk=(abs(Vmeas)/Vnom);%(Vmeas/Vnom)
switch LoadType  % 1 for Constant Z, 2 for Constant I and 3 for Constant P, 
    case 1
        Kz=1;
    case 2
        if Vk >= Vlim % convert to Constant Z load due to voltage violation
            Ki=1;
        else
            Kz=1;
        end
    case 3
        if Vk >= Vlim % convert to Constant Z load due to voltage violation
           Kp=1;
        else
            Kz=1;
        end          
 
end
Pl=Pnom *((Kz*Vk*Vk)+(Ki*Vk)+(Kp));
Ql=Qnom *((Kz*Vk*Vk)+(Ki*Vk)+(Kp));
% Net Injected Curent.
% j=sqrt(-1);
Iinj = conj((Pl+j*Ql)/Vmeas);
Iinjinst =abs(Iinj)*sqrt(2)*sin(2*fnom*pi*clock + angle(Iinj)+Ddel);
yt=Iinj;

== matlab function IEEE123bus_v2019b_Discrete_ZIPload/77 Y PQ/Embedded MATLAB Function ==
  data: Iinjinst output; Vmeas input; LoadType parameter; Vnom parameter; Pnom parameter; Qnom parameter; Vlim parameter; fnom parameter; clock input; Ddel input
%Single Phase ZIP Load
%Author: Arun Suresh, University of North Carolina, Charlotte
%Iinj=((Pnom+jQnom)/Vmeas)'
function Iinjinst = InjectedCurrent(Vmeas,LoadType,Vnom,Pnom,Qnom,Vlim,fnom,clock,Ddel)
% Calculate Pl and Ql.
%  Vmeas=1.2303e+03 + 1.9328e+03i;
Kz=0;Ki=0;Kp=0;
Vk=(abs(Vmeas)/Vnom);%(Vmeas/Vnom)
switch LoadType  % 1 for Constant Z, 2 for Constant I and 3 for Constant P, 
    case 1
        Kz=1;
    case 2
        if Vk >= Vlim % convert to Constant Z load due to voltage violation
            Ki=1;
        else
            Kz=1;
        end
    case 3
        if Vk >= Vlim % convert to Constant Z load due to voltage violation
           Kp=1;
        else
            Kz=1;
        end          
 
end
Pl=Pnom *((Kz*Vk*Vk)+(Ki*Vk)+(Kp));
Ql=Qnom *((Kz*Vk*Vk)+(Ki*Vk)+(Kp));
% Net Injected Curent.
% j=sqrt(-1);
Iinj = conj((Pl+j*Ql)/Vmeas);
Iinjinst =abs(Iinj)*sqrt(2)*sin(2*fnom*pi*clock + angle(Iinj)+Ddel);
yt=Iinj;

== matlab function IEEE123bus_v2019b_Discrete_ZIPload/79 Y Z/Embedded MATLAB Function ==
  data: Iinjinst output; Vmeas input; LoadType parameter; Vnom parameter; Pnom parameter; Qnom parameter; Vlim parameter; fnom parameter; clock input; Ddel input
%Single Phase ZIP Load
%Author: Arun Suresh, University of North Carolina, Charlotte
%Iinj=((Pnom+jQnom)/Vmeas)'
function Iinjinst = InjectedCurrent(Vmeas,LoadType,Vnom,Pnom,Qnom,Vlim,fnom,clock,Ddel)
% Calculate Pl and Ql.
%  Vmeas=1.2303e+03 + 1.9328e+03i;
Kz=0;Ki=0;Kp=0;
Vk=(abs(Vmeas)/Vnom);%(Vmeas/Vnom)
switch LoadType  % 1 for Constant Z, 2 for Constant I and 3 for Constant P, 
    case 1
        Kz=1;
    case 2
        if Vk >= Vlim % convert to Constant Z load due to voltage violation
            Ki=1;
        else
            Kz=1;
        end
    case 3
        if Vk >= Vlim % convert to Constant Z load due to voltage violation
           Kp=1;
        else
            Kz=1;
        end          
 
end
Pl=Pnom *((Kz*Vk*Vk)+(Ki*Vk)+(Kp));
Ql=Qnom *((Kz*Vk*Vk)+(Ki*Vk)+(Kp));
% Net Injected Curent.
% j=sqrt(-1);
Iinj = conj((Pl+j*Ql)/Vmeas);
Iinjinst =abs(Iinj)*sqrt(2)*sin(2*fnom*pi*clock + angle(Iinj)+Ddel);
yt=Iinj;

== matlab function IEEE123bus_v2019b_Discrete_ZIPload/80 Y PQ/Embedded MATLAB Function ==
  data: Iinjinst output; Vmeas input; LoadType parameter; Vnom parameter; Pnom parameter; Qnom parameter; Vlim parameter; fnom parameter; clock input; Ddel input
%Single Phase ZIP Load
%Author: Arun Suresh, University of North Carolina, Charlotte
%Iinj=((Pnom+jQnom)/Vmeas)'
function Iinjinst = InjectedCurrent(Vmeas,LoadType,Vnom,Pnom,Qnom,Vlim,fnom,clock,Ddel)
% Calculate Pl and Ql.
%  Vmeas=1.2303e+03 + 1.9328e+03i;
Kz=0;Ki=0;Kp=0;
Vk=(abs(Vmeas)/Vnom);%(Vmeas/Vnom)
switch LoadType  % 1 for Constant Z, 2 for Constant I and 3 for Constant P, 
    case 1
        Kz=1;
    case 2
        if Vk >= Vlim % convert to Constant Z load due to voltage violation
            Ki=1;
        else
            Kz=1;
        end
    case 3
        if Vk >= Vlim % convert to Constant Z load due to voltage violation
           Kp=1;
        else
            Kz=1;
        end          
 
end
Pl=Pnom *((Kz*Vk*Vk)+(Ki*Vk)+(Kp));
Ql=Qnom *((Kz*Vk*Vk)+(Ki*Vk)+(Kp));
% Net Injected Curent.
% j=sqrt(-1);
Iinj = conj((Pl+j*Ql)/Vmeas);
Iinjinst =abs(Iinj)*sqrt(2)*sin(2*fnom*pi*clock + angle(Iinj)+Ddel);
yt=Iinj;

== matlab function IEEE123bus_v2019b_Discrete_ZIPload/84 Y PQ/Embedded MATLAB Function ==
  data: Iinjinst output; Vmeas input; LoadType parameter; Vnom parameter; Pnom parameter; Qnom parameter; Vlim parameter; fnom parameter; clock input; Ddel input
%Single Phase ZIP Load
%Author: Arun Suresh, University of North Carolina, Charlotte
%Iinj=((Pnom+jQnom)/Vmeas)'
function Iinjinst = InjectedCurrent(Vmeas,LoadType,Vnom,Pnom,Qnom,Vlim,fnom,clock,Ddel)
% Calculate Pl and Ql.
%  Vmeas=1.2303e+03 + 1.9328e+03i;
Kz=0;Ki=0;Kp=0;
Vk=(abs(Vmeas)/Vnom);%(Vmeas/Vnom)
switch LoadType  % 1 for Constant Z, 2 for Constant I and 3 for Constant P, 
    case 1
        Kz=1;
    case 2
        if Vk >= Vlim % convert to Constant Z load due to voltage violation
            Ki=1;
        else
            Kz=1;
        end
    case 3
        if Vk >= Vlim % convert to Constant Z load due to voltage violation
           Kp=1;
        else
            Kz=1;
        end          
 
end
Pl=Pnom *((Kz*Vk*Vk)+(Ki*Vk)+(Kp));
Ql=Qnom *((Kz*Vk*Vk)+(Ki*Vk)+(Kp));
% Net Injected Curent.
% j=sqrt(-1);
Iinj = conj((Pl+j*Ql)/Vmeas);
Iinjinst =abs(Iinj)*sqrt(2)*sin(2*fnom*pi*clock + angle(Iinj)+Ddel);
yt=Iinj;

== matlab function IEEE123bus_v2019b_Discrete_ZIPload/85 Y PQ/Embedded MATLAB Function ==
  data: Iinjinst output; Vmeas input; LoadType parameter; Vnom parameter; Pnom parameter; Qnom parameter; Vlim parameter; fnom parameter; clock input; Ddel input
%Single Phase ZIP Load
%Author: Arun Suresh, University of North Carolina, Charlotte
%Iinj=((Pnom+jQnom)/Vmeas)'
function Iinjinst = InjectedCurrent(Vmeas,LoadType,Vnom,Pnom,Qnom,Vlim,fnom,clock,Ddel)
% Calculate Pl and Ql.
%  Vmeas=1.2303e+03 + 1.9328e+03i;
Kz=0;Ki=0;Kp=0;
Vk=(abs(Vmeas)/Vnom);%(Vmeas/Vnom)
switch LoadType  % 1 for Constant Z, 2 for Constant I and 3 for Constant P, 
    case 1
        Kz=1;
    case 2
        if Vk >= Vlim % convert to Constant Z load due to voltage violation
            Ki=1;
        else
            Kz=1;
        end
    case 3
        if Vk >= Vlim % convert to Constant Z load due to voltage violation
           Kp=1;
        else
            Kz=1;
        end          
 
end
Pl=Pnom *((Kz*Vk*Vk)+(Ki*Vk)+(Kp));
Ql=Qnom *((Kz*Vk*Vk)+(Ki*Vk)+(Kp));
% Net Injected Curent.
% j=sqrt(-1);
Iinj = conj((Pl+j*Ql)/Vmeas);
Iinjinst =abs(Iinj)*sqrt(2)*sin(2*fnom*pi*clock + angle(Iinj)+Ddel);
yt=Iinj;

== matlab function IEEE123bus_v2019b_Discrete_ZIPload/83 Y PQ/Embedded MATLAB Function ==
  data: Iinjinst output; Vmeas input; LoadType parameter; Vnom parameter; Pnom parameter; Qnom parameter; Vlim parameter; fnom parameter; clock input; Ddel input
%Single Phase ZIP Load
%Author: Arun Suresh, University of North Carolina, Charlotte
%Iinj=((Pnom+jQnom)/Vmeas)'
function Iinjinst = InjectedCurrent(Vmeas,LoadType,Vnom,Pnom,Qnom,Vlim,fnom,clock,Ddel)
% Calculate Pl and Ql.
%  Vmeas=1.2303e+03 + 1.9328e+03i;
Kz=0;Ki=0;Kp=0;
Vk=(abs(Vmeas)/Vnom);%(Vmeas/Vnom)
switch LoadType  % 1 for Constant Z, 2 for Constant I and 3 for Constant P, 
    case 1
        Kz=1;
    case 2
        if Vk >= Vlim % convert to Constant Z load due to voltage violation
            Ki=1;
        else
            Kz=1;
        end
    case 3
        if Vk >= Vlim % convert to Constant Z load due to voltage violation
           Kp=1;
        else
            Kz=1;
        end          
 
end
Pl=Pnom *((Kz*Vk*Vk)+(Ki*Vk)+(Kp));
Ql=Qnom *((Kz*Vk*Vk)+(Ki*Vk)+(Kp));
% Net Injected Curent.
% j=sqrt(-1);
Iinj = conj((Pl+j*Ql)/Vmeas);
Iinjinst =abs(Iinj)*sqrt(2)*sin(2*fnom*pi*clock + angle(Iinj)+Ddel);
yt=Iinj;

== matlab function IEEE123bus_v2019b_Discrete_ZIPload/82 Y PQ/Embedded MATLAB Function ==
  data: Iinjinst output; Vmeas input; LoadType parameter; Vnom parameter; Pnom parameter; Qnom parameter; Vlim parameter; fnom parameter; clock input; Ddel input
%Single Phase ZIP Load
%Author: Arun Suresh, University of North Carolina, Charlotte
%Iinj=((Pnom+jQnom)/Vmeas)'
function Iinjinst = InjectedCurrent(Vmeas,LoadType,Vnom,Pnom,Qnom,Vlim,fnom,clock,Ddel)
% Calculate Pl and Ql.
%  Vmeas=1.2303e+03 + 1.9328e+03i;
Kz=0;Ki=0;Kp=0;
Vk=(abs(Vmeas)/Vnom);%(Vmeas/Vnom)
switch LoadType  % 1 for Constant Z, 2 for Constant I and 3 for Constant P, 
    case 1
        Kz=1;
    case 2
        if Vk >= Vlim % convert to Constant Z load due to voltage violation
            Ki=1;
        else
            Kz=1;
        end
    case 3
        if Vk >= Vlim % convert to Constant Z load due to voltage violation
           Kp=1;
        else
            Kz=1;
        end          
 
end
Pl=Pnom *((Kz*Vk*Vk)+(Ki*Vk)+(Kp));
Ql=Qnom *((Kz*Vk*Vk)+(Ki*Vk)+(Kp));
% Net Injected Curent.
% j=sqrt(-1);
Iinj = conj((Pl+j*Ql)/Vmeas);
Iinjinst =abs(Iinj)*sqrt(2)*sin(2*fnom*pi*clock + angle(Iinj)+Ddel);
yt=Iinj;

== matlab function IEEE123bus_v2019b_Discrete_ZIPload/86 Y PQ/Embedded MATLAB Function ==
  data: Iinjinst output; Vmeas input; LoadType parameter; Vnom parameter; Pnom parameter; Qnom parameter; Vlim parameter; fnom parameter; clock input; Ddel input
%Single Phase ZIP Load
%Author: Arun Suresh, University of North Carolina, Charlotte
%Iinj=((Pnom+jQnom)/Vmeas)'
function Iinjinst = InjectedCurrent(Vmeas,LoadType,Vnom,Pnom,Qnom,Vlim,fnom,clock,Ddel)
% Calculate Pl and Ql.
%  Vmeas=1.2303e+03 + 1.9328e+03i;
Kz=0;Ki=0;Kp=0;
Vk=(abs(Vmeas)/Vnom);%(Vmeas/Vnom)
switch LoadType  % 1 for Constant Z, 2 for Constant I and 3 for Constant P, 
    case 1
        Kz=1;
    case 2
        if Vk >= Vlim % convert to Constant Z load due to voltage violation
            Ki=1;
        else
            Kz=1;
        end
    case 3
        if Vk >= Vlim % convert to Constant Z load due to voltage violation
           Kp=1;
        else
            Kz=1;
        end          
 
end
Pl=Pnom *((Kz*Vk*Vk)+(Ki*Vk)+(Kp));
Ql=Qnom *((Kz*Vk*Vk)+(Ki*Vk)+(Kp));
% Net Injected Curent.
% j=sqrt(-1);
Iinj = conj((Pl+j*Ql)/Vmeas);
Iinjinst =abs(Iinj)*sqrt(2)*sin(2*fnom*pi*clock + angle(Iinj)+Ddel);
yt=Iinj;

== matlab function IEEE123bus_v2019b_Discrete_ZIPload/76 DI/Embedded MATLAB Function1 ==
  data: Iinjinst output; Vmeas input; LoadType parameter; Vnom parameter; Pnom parameter; Qnom parameter; Vlim parameter; fnom parameter; clock input; Ddel input
%Three Phase Delta ZIP Load
%Author: Arun Suresh, University of North Carolina, Charlotte
%Pl=Pnom(Kz*(Vmeas/Vnom)^2+Ki(Vmeas/Vnom)+Kp), nom-nominal value,meas-measured value
%Ql=Qnom(Kz*(Vmeas/Vnom)^2+Ki(Vmeas/Vnom)+Kp), nom-nominal value,meas-measured value
%Iinj=((Pl+jQl)/Vmeas)'
function Iinjinst  = InjectedCurrent(Vmeas,LoadType,Vnom,Pnom,Qnom,Vlim,fnom,clock,Ddel)
% Calculate Pl and Ql.
Kz=0;Ki=0;Kp=0;
Vk=abs(Vmeas/(Vnom));%(Vmeas/Vnom)
switch LoadType  % 1 for Constant Z, 2 for Constant I and 3 for Constant P, 
    case 1
        Kz=1;
    case 2
        if Vk >= Vlim % convert to Constant Z load due to voltage violation
            Ki=1;
        else
            Kz=1;
        end
    case 3
        if Vk >= Vlim % convert to Constant Z load due to voltage violation
           Kp=1;
        else
            Kz=1;
        end          
 
end
Pl=Pnom'.*((Kz*Vk.*Vk)+(Ki*Vk)+(Kp));
Ql=Qnom'.*((Kz*Vk.*Vk)+(Ki*Vk)+(Kp));
% Net Injected Curent.
% j=sqrt(-1);
Iinj = conj((Pl+j*Ql)./Vmeas);
Iinjinsta =abs(Iinj(1))*sqrt(2)*sin(2*fnom*pi*clock + angle(Iinj(1))+Ddel(1));
Iinjinstb =abs(Iinj(2))*sqrt(2)*sin(2*fnom*pi*clock + angle(Iinj(2))+Ddel(2));
Iinjinstc =abs(Iinj(3))*sqrt(2)*sin(2*fnom*pi*clock + angle(Iinj(3))+Ddel(3));
Iinjinst=[Iinjinsta  Iinjinstb  Iinjinstc]';

== matlab function IEEE123bus_v2019b_Discrete_ZIPload/88 Y PQ/Embedded MATLAB Function ==
  data: Iinjinst output; Vmeas input; LoadType parameter; Vnom parameter; Pnom parameter; Qnom parameter; Vlim parameter; fnom parameter; clock input; Ddel input
%Single Phase ZIP Load
%Author: Arun Suresh, University of North Carolina, Charlotte
%Iinj=((Pnom+jQnom)/Vmeas)'
function Iinjinst = InjectedCurrent(Vmeas,LoadType,Vnom,Pnom,Qnom,Vlim,fnom,clock,Ddel)
% Calculate Pl and Ql.
%  Vmeas=1.2303e+03 + 1.9328e+03i;
Kz=0;Ki=0;Kp=0;
Vk=(abs(Vmeas)/Vnom);%(Vmeas/Vnom)
switch LoadType  % 1 for Constant Z, 2 for Constant I and 3 for Constant P, 
    case 1
        Kz=1;
    case 2
        if Vk >= Vlim % convert to Constant Z load due to voltage violation
            Ki=1;
        else
            Kz=1;
        end
    case 3
        if Vk >= Vlim % convert to Constant Z load due to voltage violation
           Kp=1;
        else
            Kz=1;
        end          
 
end
Pl=Pnom *((Kz*Vk*Vk)+(Ki*Vk)+(Kp));
Ql=Qnom *((Kz*Vk*Vk)+(Ki*Vk)+(Kp));
% Net Injected Curent.
% j=sqrt(-1);
Iinj = conj((Pl+j*Ql)/Vmeas);
Iinjinst =abs(Iinj)*sqrt(2)*sin(2*fnom*pi*clock + angle(Iinj)+Ddel);
yt=Iinj;

== matlab function IEEE123bus_v2019b_Discrete_ZIPload/87 Y PQ/Embedded MATLAB Function ==
  data: Iinjinst output; Vmeas input; LoadType parameter; Vnom parameter; Pnom parameter; Qnom parameter; Vlim parameter; fnom parameter; clock input; Ddel input
%Single Phase ZIP Load
%Author: Arun Suresh, University of North Carolina, Charlotte
%Iinj=((Pnom+jQnom)/Vmeas)'
function Iinjinst = InjectedCurrent(Vmeas,LoadType,Vnom,Pnom,Qnom,Vlim,fnom,clock,Ddel)
% Calculate Pl and Ql.
%  Vmeas=1.2303e+03 + 1.9328e+03i;
Kz=0;Ki=0;Kp=0;
Vk=(abs(Vmeas)/Vnom);%(Vmeas/Vnom)
switch LoadType  % 1 for Constant Z, 2 for Constant I and 3 for Constant P, 
    case 1
        Kz=1;
    case 2
        if Vk >= Vlim % convert to Constant Z load due to voltage violation
            Ki=1;
        else
            Kz=1;
        end
    case 3
        if Vk >= Vlim % convert to Constant Z load due to voltage violation
           Kp=1;
        else
            Kz=1;
        end          
 
end
Pl=Pnom *((Kz*Vk*Vk)+(Ki*Vk)+(Kp));
Ql=Qnom *((Kz*Vk*Vk)+(Ki*Vk)+(Kp));
% Net Injected Curent.
% j=sqrt(-1);
Iinj = conj((Pl+j*Ql)/Vmeas);
Iinjinst =abs(Iinj)*sqrt(2)*sin(2*fnom*pi*clock + angle(Iinj)+Ddel);
yt=Iinj;

== matlab function IEEE123bus_v2019b_Discrete_ZIPload/90 Y I/Embedded MATLAB Function ==
  data: Iinjinst output; Vmeas input; LoadType parameter; Vnom parameter; Pnom parameter; Qnom parameter; Vlim parameter; fnom parameter; clock input; Ddel input
%Single Phase ZIP Load
%Author: Arun Suresh, University of North Carolina, Charlotte
%Iinj=((Pnom+jQnom)/Vmeas)'
function Iinjinst = InjectedCurrent(Vmeas,LoadType,Vnom,Pnom,Qnom,Vlim,fnom,clock,Ddel)
% Calculate Pl and Ql.
%  Vmeas=1.2303e+03 + 1.9328e+03i;
Kz=0;Ki=0;Kp=0;
Vk=(abs(Vmeas)/Vnom);%(Vmeas/Vnom)
switch LoadType  % 1 for Constant Z, 2 for Constant I and 3 for Constant P, 
    case 1
        Kz=1;
    case 2
        if Vk >= Vlim % convert to Constant Z load due to voltage violation
            Ki=1;
        else
            Kz=1;
        end
    case 3
        if Vk >= Vlim % convert to Constant Z load due to voltage violation
           Kp=1;
        else
            Kz=1;
        end          
 
end
Pl=Pnom *((Kz*Vk*Vk)+(Ki*Vk)+(Kp));
Ql=Qnom *((Kz*Vk*Vk)+(Ki*Vk)+(Kp));
% Net Injected Curent.
% j=sqrt(-1);
Iinj = conj((Pl+j*Ql)/Vmeas);
Iinjinst =abs(Iinj)*sqrt(2)*sin(2*fnom*pi*clock + angle(Iinj)+Ddel);
yt=Iinj;

== matlab function IEEE123bus_v2019b_Discrete_ZIPload/92 Y PQ/Embedded MATLAB Function ==
  data: Iinjinst output; Vmeas input; LoadType parameter; Vnom parameter; Pnom parameter; Qnom parameter; Vlim parameter; fnom parameter; clock input; Ddel input
%Single Phase ZIP Load
%Author: Arun Suresh, University of North Carolina, Charlotte
%Iinj=((Pnom+jQnom)/Vmeas)'
function Iinjinst = InjectedCurrent(Vmeas,LoadType,Vnom,Pnom,Qnom,Vlim,fnom,clock,Ddel)
% Calculate Pl and Ql.
%  Vmeas=1.2303e+03 + 1.9328e+03i;
Kz=0;Ki=0;Kp=0;
Vk=(abs(Vmeas)/Vnom);%(Vmeas/Vnom)
switch LoadType  % 1 for Constant Z, 2 for Constant I and 3 for Constant P, 
    case 1
        Kz=1;
    case 2
        if Vk >= Vlim % convert to Constant Z load due to voltage violation
            Ki=1;
        else
            Kz=1;
        end
    case 3
        if Vk >= Vlim % convert to Constant Z load due to voltage violation
           Kp=1;
        else
            Kz=1;
        end          
 
end
Pl=Pnom *((Kz*Vk*Vk)+(Ki*Vk)+(Kp));
Ql=Qnom *((Kz*Vk*Vk)+(Ki*Vk)+(Kp));
% Net Injected Curent.
% j=sqrt(-1);
Iinj = conj((Pl+j*Ql)/Vmeas);
Iinjinst =abs(Iinj)*sqrt(2)*sin(2*fnom*pi*clock + angle(Iinj)+Ddel);
yt=Iinj;

== matlab function IEEE123bus_v2019b_Discrete_ZIPload/94 Y PQ/Embedded MATLAB Function ==
  data: Iinjinst output; Vmeas input; LoadType parameter; Vnom parameter; Pnom parameter; Qnom parameter; Vlim parameter; fnom parameter; clock input; Ddel input
%Single Phase ZIP Load
%Author: Arun Suresh, University of North Carolina, Charlotte
%Iinj=((Pnom+jQnom)/Vmeas)'
function Iinjinst = InjectedCurrent(Vmeas,LoadType,Vnom,Pnom,Qnom,Vlim,fnom,clock,Ddel)
% Calculate Pl and Ql.
%  Vmeas=1.2303e+03 + 1.9328e+03i;
Kz=0;Ki=0;Kp=0;
Vk=(abs(Vmeas)/Vnom);%(Vmeas/Vnom)
switch LoadType  % 1 for Constant Z, 2 for Constant I and 3 for Constant P, 
    case 1
        Kz=1;
    case 2
        if Vk >= Vlim % convert to Constant Z load due to voltage violation
            Ki=1;
        else
            Kz=1;
        end
    case 3
        if Vk >= Vlim % convert to Constant Z load due to voltage violation
           Kp=1;
        else
            Kz=1;
        end          
 
end
Pl=Pnom *((Kz*Vk*Vk)+(Ki*Vk)+(Kp));
Ql=Qnom *((Kz*Vk*Vk)+(Ki*Vk)+(Kp));
% Net Injected Curent.
% j=sqrt(-1);
Iinj = conj((Pl+j*Ql)/Vmeas);
Iinjinst =abs(Iinj)*sqrt(2)*sin(2*fnom*pi*clock + angle(Iinj)+Ddel);
yt=Iinj;
